simulink model "TIE2019Simulation"  (R2016b)
settings: Solver=FixedStepAuto  StartTime=0.0  StopTime=100  FixedStep=0.01  RelTol=1e-3
InitFcn:
  | Disturbance_rotor_payload_ini;
StopFcn:
  | PlotResults;
values from neighbouring files (symbols this model uses):
  b1 = 220    [Disturbance_rotor_payload_ini.m]
  b2 = 110    [Disturbance_rotor_payload_ini.m]
  c_v = 1    [Disturbance_rotor_payload_ini.m]
  c_x = 1    [Disturbance_rotor_payload_ini.m]
  delta_W = 0*n    [Disturbance_rotor_payload_ini.m]
  g_I = [0 0 9.8]'    [Disturbance_rotor_payload_ini.m]
  invJ_B1 = inv(J)    [Disturbance_rotor_payload_ini.m]
  J = [2 0.3 -0.5;0.3 1 0.2;-0.5 0.2 3]*10^-2    [Disturbance_rotor_payload_ini.m]
  k = 0.6    [Disturbance_rotor_payload_ini.m]
  k_e = 15    [Disturbance_rotor_payload_ini.m]
  K_omega = 1*eye(3)    [Disturbance_rotor_payload_ini.m]
  K_q = 100    [Disturbance_rotor_payload_ini.m]
  K_R = 1*eye(3)    [Disturbance_rotor_payload_ini.m]
  k_v = 15    [Disturbance_rotor_payload_ini.m]
  L = 2    [Disturbance_rotor_payload_ini.m]
  Lambda_initalB01 = angle2quat(initial_Euler(3),initial_Euler(2),initial_Euler(1))    [Disturbance_rotor_payload_ini.m]
  lambda_p = 0.2    [Disturbance_rotor_payload_ini.m]
  lambda_q = 0.3    [Disturbance_rotor_payload_ini.m]
  lambda_theta = 1    [Disturbance_rotor_payload_ini.m]
  lambda_x = 1/20    (= 0.05)    [Disturbance_rotor_payload_ini.m]
  m_p = 2    [Disturbance_rotor_payload_ini.m]
  m_q = 2    [Disturbance_rotor_payload_ini.m]
  mid_point = (mid_point1+mid_point2)/2    [Disturbance_rotor_payload_ini.m]
  n = [n;0]    [Disturbance_rotor_payload_ini.m]
  n_ = n_/norm(n_)    [Disturbance_rotor_payload_ini.m]
  omega_b01 = [0.1 0.3 0]'    [Disturbance_rotor_payload_ini.m]
  sin_W = -5    [Disturbance_rotor_payload_ini.m]
  U_initial = [y_dot_initial;v_q]    [Disturbance_rotor_payload_ini.m]
  W_0 = (m_p+m_q)*v_q + m_p*B0*y_dot_initial    [Disturbance_rotor_payload_ini.m]
  W_p = [-3 3 -0.5]'    [Disturbance_rotor_payload_ini.m]
  W_q = [-5 4 -0.3]'    [Disturbance_rotor_payload_ini.m]
  waypoint_n = [n1 n2 n3 n4 n5]    [Disturbance_rotor_payload_ini.m]
  waypoint_p = [P1 P2 P3 P4 P5]    [Disturbance_rotor_payload_ini.m]
  waypoint_v = [v1 v2 v3 v4 v5]'    [Disturbance_rotor_payload_ini.m]
  X_initial = [0 0 0]'    [Disturbance_rotor_payload_ini.m]
  y_inital = [0.02 -0.02]'    [Disturbance_rotor_payload_ini.m]
libraries: aerolibtransform2 x4, dspmtrx3 x2, aerolibutil x2, dspinverses x2
(part 1 of 2)
settings Model: Creator=arthus  LastModifiedBy=longh

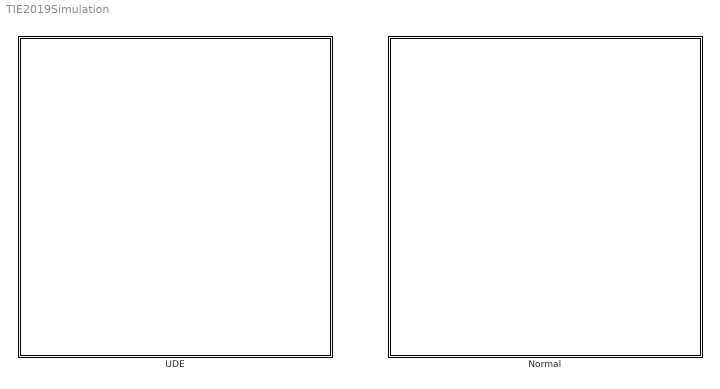
== system TIE2019Simulation ==
  Normal : Subsystem
  UDE : Subsystem
  wires:
  ? -> ?

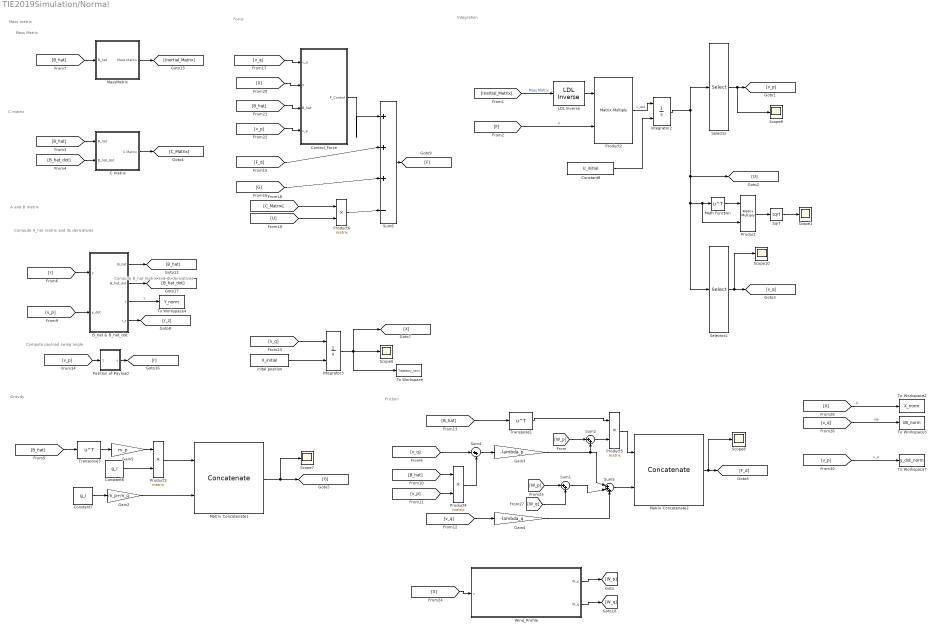
== system TIE2019Simulation/Normal ==
  note: Friction
  note: Gravity
  note: C matrix
  note: Force
  note: A and B matrix
  note: Mass matrix
  note: Mass Matrix
  note: Compute B_hat matrix and its derivatives
  note: Compute A_hat matrix and its derivatives
  note: Integration
  note: Compute payload swing angle
  note: X
  B_hat & B_hat_dot : Subsystem
  C matrix : Subsystem
  Constant6 : Constant  Value=g_I  VectorParams1D=off
  Constant7 : Constant  Value=g_I  VectorParams1D=off
  Constant8 : Constant  Value=U_initial  VectorParams1D=off
  Control_Force : Subsystem
  Gain2 : Gain  Gain=m_p+m_q
  Gain3 : Gain  Gain=-lambda_p
  Gain4 : Gain  Gain=-lambda_q
  Gain5 : Gain  Gain=m_p
  Integrator2 : Integrator  InitialConditionSource=external  InitialCondition=U_initial
  Integrator3 : Integrator  InitialConditionSource=external
  LDL Inverse : dspinverses/LDL Inverse  errmode=Error
  MassMatrix : Subsystem
  Math Function : Math  Operator=transpose  SaturateOnIntegerOverflow=on
  Matrix Concatenate1 : Concatenate  Mode=Multidimensional array
  Matrix Concatenate2 : Concatenate  Mode=Multidimensional array
  Position of Payload : Subsystem
  Product{,3..6} (5 alike) : Product  Multiplication=Matrix(*)
  Product2 : Product  Multiplication=Matrix(*)  RndMeth=Zero
  Scope{1,6..10} (6 alike) : Scope
  Selector : Selector  InputPortWidth=5  IndexOptions=Index vector (dialog)  Indices=[1 2]  OutputSizes=1
  Selector2 : Selector  InputPortWidth=5  IndexOptions=Index vector (dialog)  Indices=[3 4 5]  OutputSizes=1
  Sqrt : Sqrt  SaturateOnIntegerOverflow=on
  Sum1 : Sum  Inputs=|++
  Sum2 : Sum  Inputs=|++
  Sum4 : Sum  Inputs=|++
  Sum5 : Sum  Inputs=|+++
  Sum6 : Sum  Inputs=|+++-
  To Workspace : ToWorkspace  VariableName=Trajectory_norm  SampleTime=-1
  To Workspace2 : ToWorkspace  VariableName=X_norm  SaveFormat=Structure With Time  SampleTime=-1
  To Workspace3 : ToWorkspace  VariableName=VB_norm  SaveFormat=Structure With Time  SampleTime=-1
  To Workspace4 : ToWorkspace  VariableName=Y_norm  SaveFormat=Structure With Time  SampleTime=-1
  To Workspace7 : ToWorkspace  VariableName=y_dot_norm  SaveFormat=Structure With Time  SampleTime=-1
  Transpose1 : Math  Operator=transpose  SaturateOnIntegerOverflow=on
  Transpose3 : Math  Operator=transpose  SaturateOnIntegerOverflow=on
  Wind_Profile : Subsystem
  inital position : Constant  Value=X_initial
  wires:
  MassMatrix/1(Mass Matrix) -> [Inertial_Matrix]
  B_hat & B_hat_dot/2(B_hat_dot) -> [B_hat_dot]
  B_hat & B_hat_dot/1(B_hat) -> [B_hat]
  [r] -> B_hat & B_hat_dot/1(y)
  [v_p] -> B_hat & B_hat_dot/2(y_dot)
  [B_hat] -> MassMatrix/1(B_hat)
  LDL Inverse/1 -> Product2/1
  [Inertial_Matrix] -> LDL Inverse/1  "Mass Matrix"
  [F] -> Product2/2  "F"
  Selector/1 -> Scope9/1, [v_p]
  Product2/1 -> Integrator2/1  "u_dot"
  Integrator2/1 -> Selector/1, [U], Product/2, Math Function/1, Selector2/1
  Selector2/1 -> Scope10/1, [v_q]
  C matrix/1(C Matrix) -> [C_Matrix]
  [B_hat] -> C matrix/1(B_hat)
  [B_hat_dot] -> C matrix/2(B_hat_dot)
  [B_hat] -> Transpose3/1
  Gain5/1 -> Product3/1
  Constant6/1 -> Product3/2
  Transpose3/1 -> Gain5/1
  Product3/1 -> Matrix Concatenate1/1
  Constant7/1 -> Gain2/1
  Gain2/1 -> Matrix Concatenate1/2
  Matrix Concatenate1/1 -> Scope7/1, [G]
  Matrix Concatenate2/1 -> Scope8/1, [F_d]
  Sum5/1 -> Matrix Concatenate2/2
  Sum4/1 -> Gain3/1
  [v_q] -> Sum4/1
  [B_hat] -> Product4/1
  [v_p] -> Product4/2
  Product4/1 -> Sum4/2
  [v_q] -> Gain4/1
  [B_hat] -> Transpose1/1
  Transpose1/1 -> Product5/1
  Product5/1 -> Matrix Concatenate2/1
  Position of Payload/1(y) -> [r]
  [v_p] -> Position of Payload/1(y_dot)
  Sum6/1 -> [F]
  Control_Force/1(F_Control) -> Sum6/1
  [F_d] -> Sum6/2
  [G] -> Sum6/3
  [C_Matrix] -> Product6/1
  [U] -> Product6/2
  Product6/1 -> Sum6/4
  inital position/1 -> Integrator3/2
  [v_q] -> Integrator3/1
  Constant8/1 -> Integrator2/2
  [v_q] -> Control_Force/1(v_q)
  [X] -> Control_Force/2(X)
  B_hat & B_hat_dot/4(r_z) -> [r_z]
  Integrator3/1 -> To Workspace/1, [X], Scope6/1
  Gain4/1 -> Sum5/3
  Sum1/1 -> Sum5/2
  Sum2/1 -> Product5/2
  Gain3/1 -> Sum2/2, Sum5/1
  [B_hat] -> Control_Force/3("B_hat ")
  [v_p] -> Control_Force/4(v_p)
  B_hat & B_hat_dot/3(Y) -> To Workspace4/1  "Y"
  [v_q] -> To Workspace3/1  "VB"
  [X] -> To Workspace2/1
  [v_p] -> To Workspace7/1  "v_p"
  Wind_Profile/1(W_p) -> [W_p]
  [W_p] -> Sum2/1
  [W_q] -> Sum1/2
  [W_p] -> Sum1/1
  Math Function/1 -> Product/1
  Product/1 -> Sqrt/1
  Sqrt/1 -> Scope1/1
  Wind_Profile/2(W_q) -> [W_q]
  [X] -> Wind_Profile/1(x)

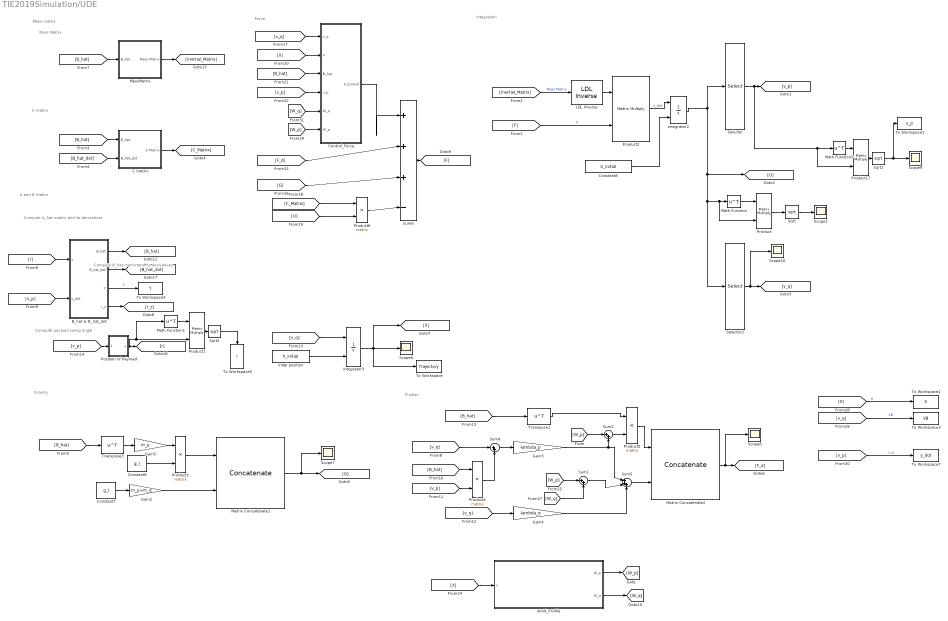
== system TIE2019Simulation/UDE ==
  note: Friction
  note: Gravity
  note: C matrix
  note: Force
  note: A and B matrix
  note: Mass matrix
  note: Mass Matrix
  note: Compute B_hat matrix and its derivatives
  note: Compute A_hat matrix and its derivatives
  note: Integration
  note: Compute payload swing angle
  note: X
  B_hat & B_hat_dot : Subsystem
  C matrix : Subsystem
  Constant6 : Constant  Value=g_I  VectorParams1D=off
  Constant7 : Constant  Value=g_I  VectorParams1D=off
  Constant8 : Constant  Value=U_initial  VectorParams1D=off
  Control_Force : Subsystem
  Gain2 : Gain  Gain=m_p+m_q
  Gain3 : Gain  Gain=-lambda_p
  Gain4 : Gain  Gain=-lambda_q
  Gain5 : Gain  Gain=m_p
  Integrator2 : Integrator  InitialConditionSource=external  InitialCondition=U_initial
  Integrator3 : Integrator  InitialConditionSource=external
  LDL Inverse : dspinverses/LDL Inverse  errmode=Error
  MassMatrix : Subsystem
  Math Function : Math  Operator=transpose  SaturateOnIntegerOverflow=on
  Math Function1 : Math  Operator=transpose  SaturateOnIntegerOverflow=on
  Math Function5 : Math  Operator=transpose  SaturateOnIntegerOverflow=on
  Matrix Concatenate1 : Concatenate  Mode=Multidimensional array
  Matrix Concatenate2 : Concatenate  Mode=Multidimensional array
  Position of Payload : Subsystem
  Product{,1,3..6,17} (7 alike) : Product  Multiplication=Matrix(*)
  Product2 : Product  Multiplication=Matrix(*)  RndMeth=Zero
  Scope{1,6..10} (6 alike) : Scope
  Selector : Selector  InputPortWidth=5  IndexOptions=Index vector (dialog)  Indices=[1 2]  OutputSizes=1
  Selector2 : Selector  InputPortWidth=5  IndexOptions=Index vector (dialog)  Indices=[3 4 5]  OutputSizes=1
  Sqrt : Sqrt  SaturateOnIntegerOverflow=on
  Sqrt1 : Sqrt  SaturateOnIntegerOverflow=on
  Sqrt2 : Sqrt  SaturateOnIntegerOverflow=on
  Sum1 : Sum  Inputs=|++
  Sum2 : Sum  Inputs=|++
  Sum4 : Sum  Inputs=|++
  Sum5 : Sum  Inputs=|+++
  Sum6 : Sum  Inputs=|+++-
  To Workspace : ToWorkspace  VariableName=Trajectory  SampleTime=-1
  To Workspace1 : ToWorkspace  VariableName=v_p  SampleTime=-1
  To Workspace2 : ToWorkspace  VariableName=X  SaveFormat=Structure With Time  SampleTime=-1
  To Workspace3 : ToWorkspace  VariableName=VB  SaveFormat=Structure With Time  SampleTime=-1
  To Workspace4 : ToWorkspace  VariableName=Y  SaveFormat=Structure With Time  SampleTime=-1
  To Workspace5 : ToWorkspace  VariableName=r  SampleTime=-1
  To Workspace7 : ToWorkspace  VariableName=y_dot  SaveFormat=Structure With Time  SampleTime=-1
  Transpose1 : Math  Operator=transpose  SaturateOnIntegerOverflow=on
  Transpose3 : Math  Operator=transpose  SaturateOnIntegerOverflow=on
  Wind_Profile : Subsystem
  inital position : Constant  Value=X_initial
  wires:
  MassMatrix/1(Mass Matrix) -> [Inertial_Matrix]
  B_hat & B_hat_dot/2(B_hat_dot) -> [B_hat_dot]
  B_hat & B_hat_dot/1(B_hat) -> [B_hat]
  [r] -> B_hat & B_hat_dot/1(y)
  [v_p] -> B_hat & B_hat_dot/2(y_dot)
  [B_hat] -> MassMatrix/1(B_hat)
  LDL Inverse/1 -> Product2/1
  [Inertial_Matrix] -> LDL Inverse/1  "Mass Matrix"
  [F] -> Product2/2  "F"
  Product2/1 -> Integrator2/1  "u_dot"
  Integrator2/1 -> Selector/1, [U], Product/2, Math Function/1, Selector2/1
  Selector2/1 -> Scope10/1, [v_q]
  C matrix/1(C Matrix) -> [C_Matrix]
  [B_hat] -> C matrix/1(B_hat)
  [B_hat_dot] -> C matrix/2(B_hat_dot)
  [B_hat] -> Transpose3/1
  Gain5/1 -> Product3/1
  Constant6/1 -> Product3/2
  Transpose3/1 -> Gain5/1
  Product3/1 -> Matrix Concatenate1/1
  Constant7/1 -> Gain2/1
  Gain2/1 -> Matrix Concatenate1/2
  Matrix Concatenate1/1 -> Scope7/1, [G]
  Matrix Concatenate2/1 -> Scope8/1, [F_d]
  Sum5/1 -> Matrix Concatenate2/2
  Sum4/1 -> Gain3/1
  [v_q] -> Sum4/1
  [B_hat] -> Product4/1
  [v_p] -> Product4/2
  Product4/1 -> Sum4/2
  [v_q] -> Gain4/1
  [B_hat] -> Transpose1/1
  Transpose1/1 -> Product5/1
  Product5/1 -> Matrix Concatenate2/1
  Position of Payload/1(y) -> Math Function1/1, Product1/2, [r]
  [v_p] -> Position of Payload/1(y_dot)
  Sum6/1 -> [F]
  Control_Force/1(F_Control) -> Sum6/1
  [F_d] -> Sum6/2
  [G] -> Sum6/3
  [C_Matrix] -> Product6/1
  [U] -> Product6/2
  Product6/1 -> Sum6/4
  inital position/1 -> Integrator3/2
  [v_q] -> Integrator3/1
  Constant8/1 -> Integrator2/2
  [v_q] -> Control_Force/1(v_q)
  [X] -> Control_Force/2(X)
  B_hat & B_hat_dot/4(r_z) -> [r_z]
  Integrator3/1 -> To Workspace/1, [X], Scope6/1
  Gain4/1 -> Sum5/3
  Sum1/1 -> Sum5/2
  Sum2/1 -> Product5/2
  Gain3/1 -> Sum2/2, Sum5/1
  [B_hat] -> Control_Force/3("B_hat ")
  [v_p] -> Control_Force/4(v_p)
  B_hat & B_hat_dot/3(Y) -> To Workspace4/1  "Y"
  [v_q] -> To Workspace3/1  "VB"
  [X] -> To Workspace2/1
  [v_p] -> To Workspace7/1  "v_p"
  Wind_Profile/1(W_p) -> [W_p]
  [W_p] -> Sum2/1
  [W_q] -> Sum1/2
  [W_p] -> Sum1/1
  Math Function/1 -> Product/1
  Product/1 -> Sqrt/1
  Sqrt/1 -> Scope1/1
  Wind_Profile/2(W_q) -> [W_q]
  [X] -> Wind_Profile/1(x)
  Selector/1 -> Math Function5/1, Product17/2, [v_p]
  Math Function5/1 -> Product17/1
  Product17/1 -> Sqrt1/1
  Sqrt1/1 -> To Workspace1/1, Scope9/1
  [W_p] -> Control_Force/6(W_p)
  [W_q] -> Control_Force/5(W_q)
  Math Function1/1 -> Product1/1
  Product1/1 -> Sqrt2/1
  Sqrt2/1 -> To Workspace5/1

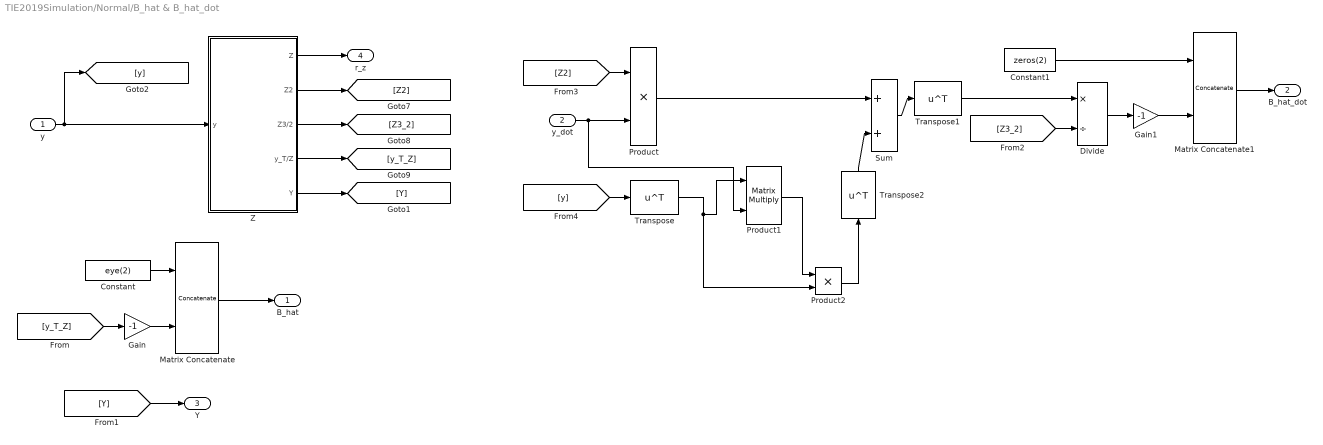
== system TIE2019Simulation/Normal/B_hat & B_hat_dot ==
  y : Inport
  y_dot : Inport  Port=2
  Constant : Constant  Value=eye(2)
  Constant1 : Constant  Value=zeros(2)
  Divide : Product  Inputs=*/
  Gain : Gain  Gain=-1
  Gain1 : Gain  Gain=-1
  Matrix Concatenate : Concatenate  Mode=Multidimensional array
  Matrix Concatenate1 : Concatenate  Mode=Multidimensional array
  Product : Product  RndMeth=Zero
  Product1 : Product  Multiplication=Matrix(*)  RndMeth=Zero
  Product2 : Product  RndMeth=Zero
  Sum : Sum
  Transpose : Math  Operator=transpose  SaturateOnIntegerOverflow=on
  Transpose1 : Math  Operator=transpose  SaturateOnIntegerOverflow=on
  Transpose2 : Math  Operator=transpose  SaturateOnIntegerOverflow=on
  Z : Subsystem
  B_hat : Outport
  B_hat_dot : Outport  Port=2
  Y : Outport  Port=3
  r_z : Outport  Port=4
  wires:
  y_dot/1 -> Product/2, Product1/2
  y/1 -> Z/1(y), [y]
  Matrix Concatenate/1 -> B_hat/1
  Matrix Concatenate1/1 -> B_hat_dot/1
  Z/1(Z) -> r_z/1
  Z/2(Z2) -> [Z2]
  Z/3(Z3/2) -> [Z3_2]
  Z/4(y_T/Z) -> [y_T_Z]
  [y_T_Z] -> Gain/1
  Constant/1 -> Matrix Concatenate/1
  Gain/1 -> Matrix Concatenate/2
  Z/5(Y) -> [Y]
  [Y] -> Y/1
  Constant1/1 -> Matrix Concatenate1/1
  [Z3_2] -> Divide/2
  Sum/1 -> Transpose1/1
  [Z2] -> Product/1
  [y] -> Transpose/1
  Transpose/1 -> Product1/1, Product2/2
  Product1/1 -> Product2/1
  Divide/1 -> Gain1/1
  Gain1/1 -> Matrix Concatenate1/2
  Product2/1 -> Transpose2/1
  Product/1 -> Sum/1
  Transpose1/1 -> Divide/1
  Transpose2/1 -> Sum/2

== system TIE2019Simulation/Normal/C matrix ==
  B_hat : Inport
  B_hat_dot : Inport  Port=2
  Constant : Constant  Value=[zeros(2,3);zeros(3)]  VectorParams1D=off
  Gain4 : Gain  Gain=m_p
  Gain5 : Gain  Gain=m_p
  Matrix Concatenate : Concatenate  Mode=Multidimensional array  ConcatenateDimension=2
  Matrix Concatenate1 : Concatenate  Mode=Multidimensional array
  Product1 : Product  Multiplication=Matrix(*)
  Transpose3 : Math  Operator=transpose  SaturateOnIntegerOverflow=on
  C Matrix : Outport
  wires:
  Matrix Concatenate/1 -> C Matrix/1
  Matrix Concatenate1/1 -> Matrix Concatenate/1
  Constant/1 -> Matrix Concatenate/2
  B_hat/1 -> Transpose3/1
  Transpose3/1 -> [B_hatT]
  Gain5/1 -> Matrix Concatenate1/1
  [B_hatT] -> Product1/1
  B_hat_dot/1 -> Gain4/1, Product1/2
  Product1/1 -> Gain5/1
  Gain4/1 -> Matrix Concatenate1/2

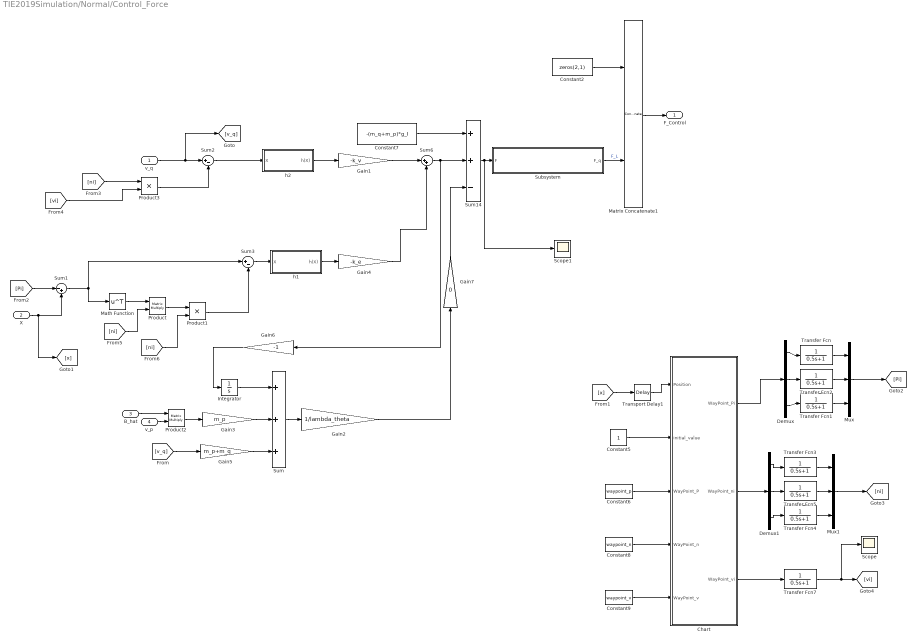
== system TIE2019Simulation/Normal/Control_Force ==
  v_q : Inport
  X : Inport  Port=2
  "B_hat " : Inport  Port=3
  v_p : Inport  Port=4
  Chart : Stateflow chart  TreatAsAtomicUnit=on
  Constant2 : Constant  Value=zeros(2,1)
  Constant5 : Constant
  Constant6 : Constant  Value=waypoint_p
  Constant7 : Constant  Value=-(m_q+m_p)*g_I  VectorParams1D=off
  Constant8 : Constant  Value=waypoint_n
  Constant9 : Constant  Value=waypoint_v
  Demux : Demux  Outputs=3
  Demux1 : Demux  Outputs=3
  Gain1 : Gain  Gain=-k_v
  Gain2 : Gain  Gain=1/lambda_theta
  Gain3 : Gain  Gain=m_p
  Gain4 : Gain  Gain=-k_e
  Gain5 : Gain  Gain=m_p+m_q
  Gain6 : Gain  Gain=-1
  Gain7 : Gain  Gain=0
  Integrator : Integrator
  Math Function : Math  Operator=transpose  SaturateOnIntegerOverflow=on
  Matrix Concatenate1 : Concatenate  Mode=Multidimensional array
  Mux : Mux  Inputs=3
  Mux1 : Mux  Inputs=3
  Product : Product  Multiplication=Matrix(*)
  Product1 : Product
  Product2 : Product  Multiplication=Matrix(*)
  Product3 : Product
  Scope : Scope
  Scope1 : Scope
  Subsystem : Subsystem
  Sum : Sum  Inputs=+++
  Sum1 : Sum  Inputs=|-+
  Sum14 : Sum  Inputs=++-
  Sum2 : Sum  Inputs=|+-
  Sum3 : Sum  Inputs=|+-
  Sum6 : Sum  Inputs=|++
  Transfer Fcn{,1..5,7} (7 alike) : TransferFcn  Denominator=[0.5 1]
  Transport Delay1 : TransportDelay  DelayTime=0.3
  h1 : Subsystem
  h2 : Subsystem
  F_Control : Outport
  wires:
  Constant2/1 -> Matrix Concatenate1/1
  X/1 -> [x], Sum1/2
  v_q/1 -> [v_q], Sum2/1
  Sum14/1 -> Scope1/1, Subsystem/1(F)
  [ni] -> Product3/1
  [Pi] -> Sum1/1
  Product3/1 -> Sum2/2
  h1/1(h(X)) -> Gain4/1
  Gain4/1 -> Sum6/2
  Sum1/1 -> Sum3/1, Math Function/1
  Math Function/1 -> Product/1
  [ni] -> Product/2
  Product/1 -> Product1/1
  [ni] -> Product1/2
  Product1/1 -> Sum3/2
  Gain1/1 -> Sum6/1
  h2/1(h(X)) -> Gain1/1
  Sum6/1 -> Gain6/1, Sum14/2
  Constant7/1 -> Sum14/1
  Gain2/1 -> Gain7/1
  Sum/1 -> Gain2/1
  "B_hat "/1 -> Product2/1
  v_p/1 -> Product2/2
  Product2/1 -> Gain3/1
  [v_q] -> Gain5/1
  Gain3/1 -> Sum/2
  Gain5/1 -> Sum/3
  Integrator/1 -> Sum/1
  Gain6/1 -> Integrator/1
  Matrix Concatenate1/1 -> F_Control/1
  Gain7/1 -> Sum14/3
  Subsystem/1(F_q) -> Matrix Concatenate1/2  "F_L"
  Constant5/1 -> Chart/2(initial_value)
  [x] -> Transport Delay1/1
  Constant6/1 -> Chart/3(WayPoint_P)
  Constant8/1 -> Chart/4(WayPoint_n)
  Constant9/1 -> Chart/5(WayPoint_v)
  [vi] -> Product3/2
  Transport Delay1/1 -> Chart/1(Position)
  Demux/3 -> Transfer Fcn1/1
  Transfer Fcn1/1 -> Mux/3
  Demux/2 -> Transfer Fcn2/1
  Transfer Fcn2/1 -> Mux/2
  Demux/1 -> Transfer Fcn/1
  Transfer Fcn/1 -> Mux/1
  Mux/1 -> [Pi]
  Chart/1(WayPoint_Pi) -> Demux/1
  Demux1/3 -> Transfer Fcn4/1
  Transfer Fcn4/1 -> Mux1/3
  Demux1/2 -> Transfer Fcn5/1
  Transfer Fcn5/1 -> Mux1/2
  Demux1/1 -> Transfer Fcn3/1
  Transfer Fcn3/1 -> Mux1/1
  Mux1/1 -> [ni]
  Chart/2(WayPoint_ni) -> Demux1/1
  Chart/3(WayPoint_vi) -> Transfer Fcn7/1
  Transfer Fcn7/1 -> Scope/1, [vi]
  Sum2/1 -> h2/1(X)
  Sum3/1 -> h1/1(X)

== system TIE2019Simulation/Normal/MassMatrix ==
  B_hat : Inport
  Constant : Constant  Value=(m_q+m_p)*eye(3)
  Gain1 : Gain  Gain=m_p
  Gain2 : Gain  Gain=m_p
  Gain3 : Gain  Gain=m_p
  Matrix Concatenate : Concatenate  Mode=Multidimensional array  ConcatenateDimension=2
  Matrix Concatenate1 : Concatenate  Mode=Multidimensional array
  Matrix Concatenate2 : Concatenate  Mode=Multidimensional array
  Product : Product  Multiplication=Matrix(*)
  Transpose3 : Math  Operator=transpose  SaturateOnIntegerOverflow=on
  Mass Matrix : Outport
  wires:
  Matrix Concatenate/1 -> Mass Matrix/1
  Matrix Concatenate1/1 -> Matrix Concatenate/1
  Matrix Concatenate2/1 -> Matrix Concatenate/2
  B_hat/1 -> [B_hat], Transpose3/1
  Transpose3/1 -> [B_hatT]
  [B_hatT] -> Product/1
  [B_hat] -> Product/2
  Product/1 -> Gain1/1
  Gain1/1 -> Matrix Concatenate1/1
  Gain2/1 -> Matrix Concatenate1/2
  [B_hat] -> Gain2/1
  Constant/1 -> Matrix Concatenate2/2
  [B_hatT] -> Gain3/1
  Gain3/1 -> Matrix Concatenate2/1

== system TIE2019Simulation/Normal/Position of Payload ==
  y_dot : Inport
  Integrator : Integrator  InitialConditionSource=external
  inital position : Constant  Value=y_inital  VectorParams1D=off
  y : Outport
  wires:
  Integrator/1 -> y/1
  y_dot/1 -> Integrator/1
  inital position/1 -> Integrator/2

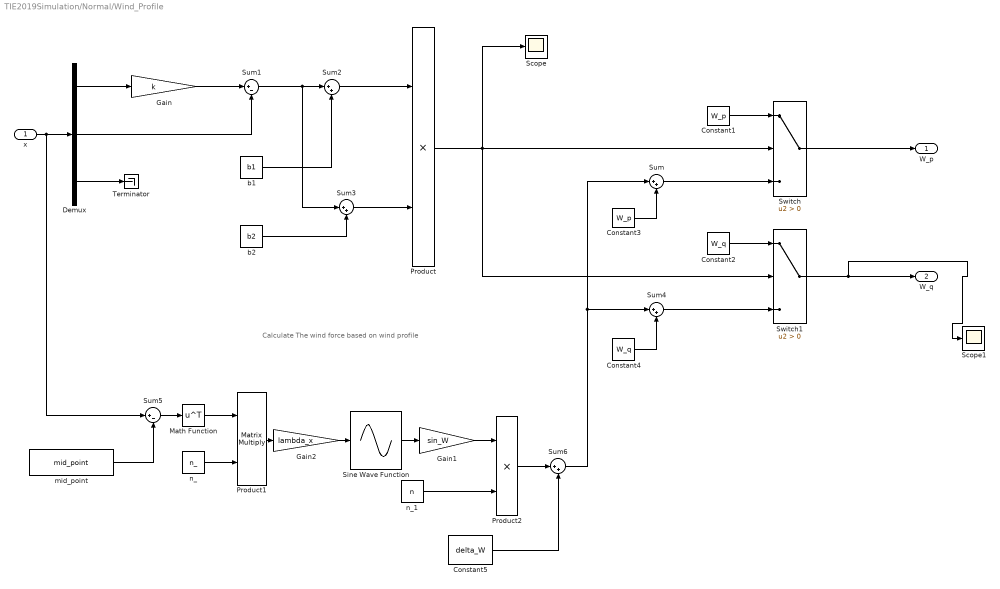
== system TIE2019Simulation/Normal/Wind_Profile ==
  note: Calculate The wind force based on wind profile
  x : Inport
  Constant1 : Constant  Value=W_p
  Constant2 : Constant  Value=W_q
  Constant3 : Constant  Value=W_p
  Constant4 : Constant  Value=W_q
  Constant5 : Constant  Value=delta_W
  Demux : Demux  Outputs=3
  Gain : Gain  Gain=k
  Gain1 : Gain  Gain=sin_W
  Gain2 : Gain  Gain=lambda_x
  Math Function : Math  Operator=transpose  SaturateOnIntegerOverflow=on
  Product : Product
  Product1 : Product  Multiplication=Matrix(*)
  Product2 : Product
  Scope : Scope
  Scope1 : Scope
  Sine Wave Function : Sin  TimeSource=Use external signal  SampleTime=0
  Sum{,2..4,6} (5 alike) : Sum  Inputs=|++
  Sum1 : Sum  Inputs=|+-
  Sum5 : Sum  Inputs=|+-
  Switch : Switch  Criteria=u2 > Threshold
  Switch1 : Switch  Criteria=u2 > Threshold
  Terminator : Terminator
  b1 : Constant  Value=b1
  b2 : Constant  Value=b2
  "mid_point " : Constant  Value=mid_point  VectorParams1D=off
  n_ : Constant  Value=n_
  n_1 : Constant  Value=n
  W_p : Outport
  W_q : Outport  Port=2
  wires:
  Demux/3 -> Terminator/1
  Demux/1 -> Gain/1
  Demux/2 -> Sum1/2
  Gain/1 -> Sum1/1
  Sum1/1 -> Sum3/1, Sum2/1
  b1/1 -> Sum2/2
  b2/1 -> Sum3/2
  Sum2/1 -> Product/1
  Sum3/1 -> Product/2
  Product/1 -> Scope/1, Switch1/2, Switch/2
  Constant2/1 -> Switch1/1
  Constant1/1 -> Switch/1
  Switch/1 -> W_p/1
  Switch1/1 -> Scope1/1, W_q/1
  Sine Wave Function/1 -> Gain1/1
  Sum/1 -> Switch/3
  Sum4/1 -> Switch1/3
  Constant3/1 -> Sum/2
  Constant4/1 -> Sum4/2
  x/1 -> Sum5/1, Demux/1
  "mid_point "/1 -> Sum5/2
  Sum5/1 -> Math Function/1
  Math Function/1 -> Product1/1
  n_/1 -> Product1/2
  Product1/1 -> Gain2/1
  Gain1/1 -> Product2/1
  n_1/1 -> Product2/2
  Gain2/1 -> Sine Wave Function/1
  Product2/1 -> Sum6/1
  Sum6/1 -> Sum4/1, Sum/1
  Constant5/1 -> Sum6/2

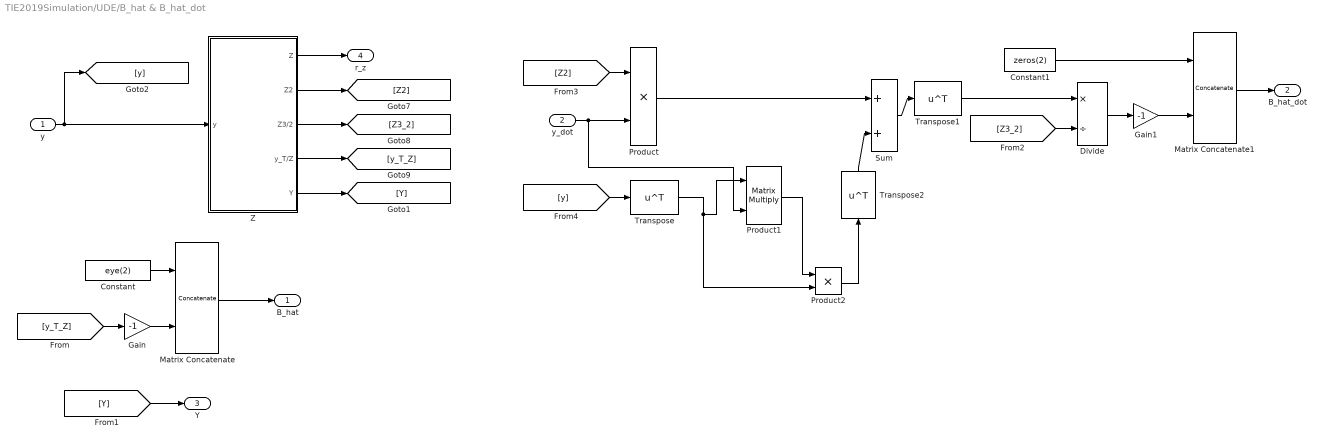
== system TIE2019Simulation/UDE/B_hat & B_hat_dot ==
  y : Inport
  y_dot : Inport  Port=2
  Constant : Constant  Value=eye(2)
  Constant1 : Constant  Value=zeros(2)
  Divide : Product  Inputs=*/
  Gain : Gain  Gain=-1
  Gain1 : Gain  Gain=-1
  Matrix Concatenate : Concatenate  Mode=Multidimensional array
  Matrix Concatenate1 : Concatenate  Mode=Multidimensional array
  Product : Product  RndMeth=Zero
  Product1 : Product  Multiplication=Matrix(*)  RndMeth=Zero
  Product2 : Product  RndMeth=Zero
  Sum : Sum
  Transpose : Math  Operator=transpose  SaturateOnIntegerOverflow=on
  Transpose1 : Math  Operator=transpose  SaturateOnIntegerOverflow=on
  Transpose2 : Math  Operator=transpose  SaturateOnIntegerOverflow=on
  Z : Subsystem
  B_hat : Outport
  B_hat_dot : Outport  Port=2
  Y : Outport  Port=3
  r_z : Outport  Port=4
  wires:
  y_dot/1 -> Product/2, Product1/2
  y/1 -> Z/1(y), [y]
  Matrix Concatenate/1 -> B_hat/1
  Matrix Concatenate1/1 -> B_hat_dot/1
  Z/1(Z) -> r_z/1
  Z/2(Z2) -> [Z2]
  Z/3(Z3/2) -> [Z3_2]
  Z/4(y_T/Z) -> [y_T_Z]
  [y_T_Z] -> Gain/1
  Constant/1 -> Matrix Concatenate/1
  Gain/1 -> Matrix Concatenate/2
  Z/5(Y) -> [Y]
  [Y] -> Y/1
  Constant1/1 -> Matrix Concatenate1/1
  [Z3_2] -> Divide/2
  Sum/1 -> Transpose1/1
  [Z2] -> Product/1
  [y] -> Transpose/1
  Transpose/1 -> Product1/1, Product2/2
  Product1/1 -> Product2/1
  Divide/1 -> Gain1/1
  Gain1/1 -> Matrix Concatenate1/2
  Product2/1 -> Transpose2/1
  Product/1 -> Sum/1
  Transpose1/1 -> Divide/1
  Transpose2/1 -> Sum/2

== system TIE2019Simulation/UDE/C matrix ==
  B_hat : Inport
  B_hat_dot : Inport  Port=2
  Constant : Constant  Value=[zeros(2,3);zeros(3)]  VectorParams1D=off
  Gain4 : Gain  Gain=m_p
  Gain5 : Gain  Gain=m_p
  Matrix Concatenate : Concatenate  Mode=Multidimensional array  ConcatenateDimension=2
  Matrix Concatenate1 : Concatenate  Mode=Multidimensional array
  Product1 : Product  Multiplication=Matrix(*)
  Transpose3 : Math  Operator=transpose  SaturateOnIntegerOverflow=on
  C Matrix : Outport
  wires:
  Matrix Concatenate/1 -> C Matrix/1
  Matrix Concatenate1/1 -> Matrix Concatenate/1
  Constant/1 -> Matrix Concatenate/2
  B_hat/1 -> Transpose3/1
  Transpose3/1 -> [B_hatT]
  Gain5/1 -> Matrix Concatenate1/1
  [B_hatT] -> Product1/1
  B_hat_dot/1 -> Gain4/1, Product1/2
  Product1/1 -> Gain5/1
  Gain4/1 -> Matrix Concatenate1/2

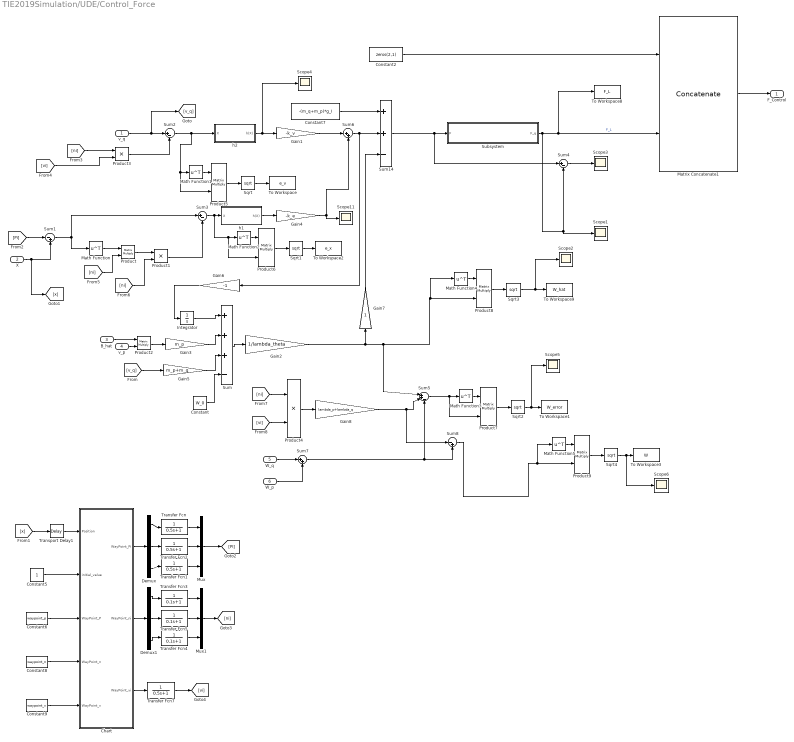
== system TIE2019Simulation/UDE/Control_Force ==
  v_q : Inport
  X : Inport  Port=2
  "B_hat " : Inport  Port=3
  v_p : Inport  Port=4
  W_q : Inport  Port=5
  W_p : Inport  Port=6
  Chart : Stateflow chart  TreatAsAtomicUnit=on
  Constant : Constant  Value=W_0  VectorParams1D=off
  Constant2 : Constant  Value=zeros(2,1)
  Constant5 : Constant
  Constant6 : Constant  Value=waypoint_p
  Constant7 : Constant  Value=-(m_q+m_p)*g_I  VectorParams1D=off
  Constant8 : Constant  Value=waypoint_n
  Constant9 : Constant  Value=waypoint_v
  Demux : Demux  Outputs=3
  Demux1 : Demux  Outputs=3
  Gain1 : Gain  Gain=-k_v
  Gain2 : Gain  Gain=1/lambda_theta
  Gain3 : Gain  Gain=m_p
  Gain4 : Gain  Gain=-k_e
  Gain5 : Gain  Gain=m_p+m_q
  Gain6 : Gain  Gain=-1
  Gain7 : Gain
  Gain8 : Gain  Gain=lambda_p+lambda_q
  Integrator : Integrator
  Math Function{,1..5} (6 alike) : Math  Operator=transpose  SaturateOnIntegerOverflow=on
  Matrix Concatenate1 : Concatenate  Mode=Multidimensional array
  Mux : Mux  Inputs=3
  Mux1 : Mux  Inputs=3
  Product{,2,5..9} (7 alike) : Product  Multiplication=Matrix(*)
  Product1 : Product
  Product3 : Product
  Product4 : Product
  Scope{1..6,11} (7 alike) : Scope
  Sqrt{,1..4} (5 alike) : Sqrt  SaturateOnIntegerOverflow=on
  Subsystem : Subsystem
  Sum : Sum  Inputs=+++-
  Sum1 : Sum  Inputs=|-+
  Sum14 : Sum  Inputs=++-
  Sum2 : Sum  Inputs=|+-
  Sum3 : Sum  Inputs=|+-
  Sum4 : Sum  Inputs=|+-
  Sum5 : Sum  Inputs=|++-
  Sum6 : Sum  Inputs=|++
  Sum7 : Sum  Inputs=|++
  Sum8 : Sum  Inputs=|-+
  To Workspace : ToWorkspace  VariableName=e_v  SampleTime=-1
  To Workspace1 : ToWorkspace  VariableName=W_error  SaveFormat=Structure With Time  SampleTime=-1
  To Workspace2 : ToWorkspace  VariableName=e_x  SampleTime=-1
  To Workspace3 : ToWorkspace  VariableName=W  SaveFormat=Structure With Time  SampleTime=-1
  To Workspace8 : ToWorkspace  VariableName=F_L  SaveFormat=Structure With Time  SampleTime=-1
  To Workspace9 : ToWorkspace  VariableName=W_hat  SaveFormat=Structure With Time  SampleTime=-1
  Transfer Fcn{,1..2,7} (4 alike) : TransferFcn  Denominator=[0.5 1]
  Transfer Fcn3 : TransferFcn  Denominator=[0.1 1]
  Transfer Fcn4 : TransferFcn  Denominator=[0.1 1]
  Transfer Fcn5 : TransferFcn  Denominator=[0.1 1]
  Transport Delay1 : TransportDelay  DelayTime=0.3
  h1 : Subsystem
  h2 : Subsystem
  F_Control : Outport
  wires:
  Constant2/1 -> Matrix Concatenate1/1
  X/1 -> [x], Sum1/2
  v_q/1 -> [v_q], Sum2/1
  Sum14/1 -> Subsystem/1(F), Sum4/1
  [ni] -> Product3/1
  [Pi] -> Sum1/1
  Product3/1 -> Sum2/2
  h1/1(h(X)) -> Gain4/1
  Gain4/1 -> Sum6/2, Scope11/1
  Sum1/1 -> Sum3/1, Math Function/1
  Math Function/1 -> Product/1
  [ni] -> Product/2
  Product/1 -> Product1/1
  [ni] -> Product1/2
  Product1/1 -> Sum3/2
  Gain1/1 -> Sum6/1
  h2/1(h(X)) -> Scope4/1, Gain1/1
  Sum6/1 -> Gain6/1, Sum14/2
  Constant7/1 -> Sum14/1
  Sum/1 -> Gain2/1
  "B_hat "/1 -> Product2/1
  v_p/1 -> Product2/2
  Product2/1 -> Gain3/1
  [v_q] -> Gain5/1
  Gain3/1 -> Sum/2
  Gain5/1 -> Sum/3
  Integrator/1 -> Sum/1
  Gain6/1 -> Integrator/1
  Matrix Concatenate1/1 -> F_Control/1
  Gain7/1 -> Sum14/3
  Subsystem/1(F_q) -> Scope1/1, Sum4/2, To Workspace8/1, Matrix Concatenate1/2  "F_L"
  Sum4/1 -> Scope3/1
  Constant5/1 -> Chart/2(initial_value)
  [x] -> Transport Delay1/1
  Constant6/1 -> Chart/3(WayPoint_P)
  Constant8/1 -> Chart/4(WayPoint_n)
  Constant9/1 -> Chart/5(WayPoint_v)
  [vi] -> Product3/2
  Transport Delay1/1 -> Chart/1(Position)
  Demux/3 -> Transfer Fcn1/1
  Transfer Fcn1/1 -> Mux/3
  Demux/2 -> Transfer Fcn2/1
  Transfer Fcn2/1 -> Mux/2
  Demux/1 -> Transfer Fcn/1
  Transfer Fcn/1 -> Mux/1
  Mux/1 -> [Pi]
  Chart/1(WayPoint_Pi) -> Demux/1
  Demux1/3 -> Transfer Fcn4/1
  Transfer Fcn4/1 -> Mux1/3
  Demux1/2 -> Transfer Fcn5/1
  Transfer Fcn5/1 -> Mux1/2
  Demux1/1 -> Transfer Fcn3/1
  Transfer Fcn3/1 -> Mux1/1
  Mux1/1 -> [ni]
  Chart/2(WayPoint_ni) -> Demux1/1
  Chart/3(WayPoint_vi) -> Transfer Fcn7/1
  Transfer Fcn7/1 -> [vi]
  [ni] -> Product4/1
  Product4/1 -> Gain8/1
  [vi] -> Product4/2
  Gain8/1 -> Sum8/1, Sum5/2
  Sum7/1 -> Sum8/2, Sum5/3
  Sum2/1 -> Product5/2, Math Function1/1, h2/1(X)
  Math Function1/1 -> Product5/1
  Product5/1 -> Sqrt/1
  Sqrt/1 -> To Workspace/1
  Sum3/1 -> Product6/2, Math Function2/1, h1/1(X)
  Math Function2/1 -> Product6/1
  Product6/1 -> Sqrt1/1
  Sum5/1 -> Product7/2, Math Function3/1
  Math Function3/1 -> Product7/1
  Product7/1 -> Sqrt2/1
  Sqrt2/1 -> Scope5/1, To Workspace1/1
  Sqrt1/1 -> To Workspace2/1
  W_q/1 -> Sum7/1
  W_p/1 -> Sum7/2
  Gain2/1 -> Math Function4/1, Product8/2, Sum5/1, Gain7/1
  Math Function4/1 -> Product8/1
  Product8/1 -> Sqrt3/1
  Sqrt3/1 -> Scope2/1, To Workspace9/1
  Sum8/1 -> Math Function5/1, Product9/2
  Math Function5/1 -> Product9/1
  Product9/1 -> Sqrt4/1
  Sqrt4/1 -> Scope6/1, To Workspace3/1
  Constant/1 -> Sum/4

== system TIE2019Simulation/UDE/MassMatrix ==
  B_hat : Inport
  Constant : Constant  Value=(m_q+m_p)*eye(3)
  Gain1 : Gain  Gain=m_p
  Gain2 : Gain  Gain=m_p
  Gain3 : Gain  Gain=m_p
  Matrix Concatenate : Concatenate  Mode=Multidimensional array  ConcatenateDimension=2
  Matrix Concatenate1 : Concatenate  Mode=Multidimensional array
  Matrix Concatenate2 : Concatenate  Mode=Multidimensional array
  Product : Product  Multiplication=Matrix(*)
  Transpose3 : Math  Operator=transpose  SaturateOnIntegerOverflow=on
  Mass Matrix : Outport
  wires:
  Matrix Concatenate/1 -> Mass Matrix/1
  Matrix Concatenate1/1 -> Matrix Concatenate/1
  Matrix Concatenate2/1 -> Matrix Concatenate/2
  B_hat/1 -> [B_hat], Transpose3/1
  Transpose3/1 -> [B_hatT]
  [B_hatT] -> Product/1
  [B_hat] -> Product/2
  Product/1 -> Gain1/1
  Gain1/1 -> Matrix Concatenate1/1
  Gain2/1 -> Matrix Concatenate1/2
  [B_hat] -> Gain2/1
  Constant/1 -> Matrix Concatenate2/2
  [B_hatT] -> Gain3/1
  Gain3/1 -> Matrix Concatenate2/1

== system TIE2019Simulation/UDE/Position of Payload ==
  y_dot : Inport
  Integrator : Integrator  InitialConditionSource=external
  inital position : Constant  Value=y_inital  VectorParams1D=off
  y : Outport
  wires:
  Integrator/1 -> y/1
  y_dot/1 -> Integrator/1
  inital position/1 -> Integrator/2

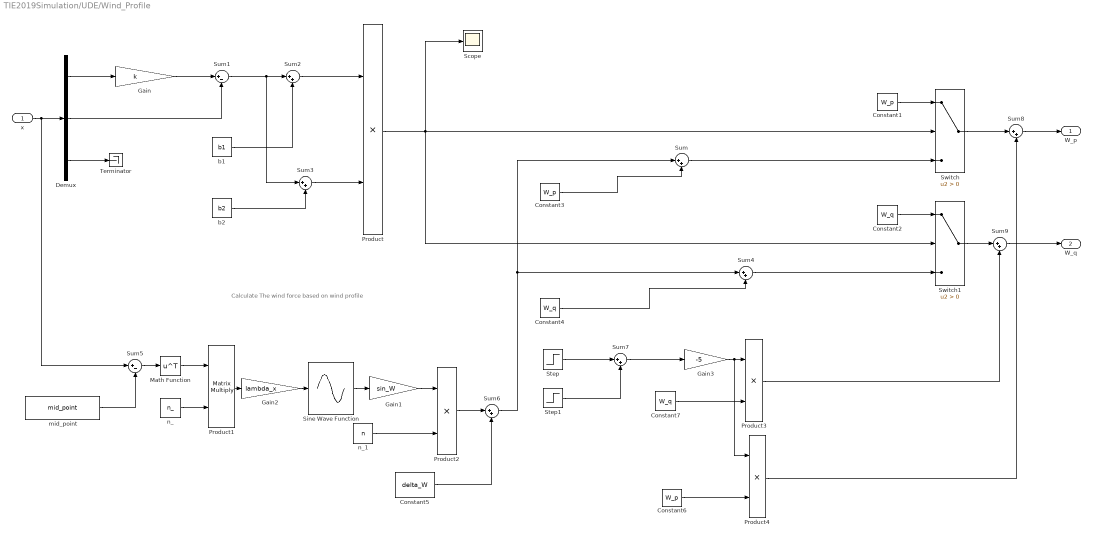
== system TIE2019Simulation/UDE/Wind_Profile ==
  note: Calculate The wind force based on wind profile
  x : Inport
  Constant1 : Constant  Value=W_p
  Constant2 : Constant  Value=W_q
  Constant3 : Constant  Value=W_p
  Constant4 : Constant  Value=W_q
  Constant5 : Constant  Value=delta_W
  Constant6 : Constant  Value=W_p
  Constant7 : Constant  Value=W_q
  Demux : Demux  Outputs=3
  Gain : Gain  Gain=k
  Gain1 : Gain  Gain=sin_W
  Gain2 : Gain  Gain=lambda_x
  Gain3 : Gain  Gain=-5
  Math Function : Math  Operator=transpose  SaturateOnIntegerOverflow=on
  Product{,2..4} (4 alike) : Product
  Product1 : Product  Multiplication=Matrix(*)
  Scope : Scope
  Sine Wave Function : Sin  TimeSource=Use external signal  SampleTime=0
  Step : Step  Time=65  SampleTime=0
  Step1 : Step  Time=67  After=-1  SampleTime=0
  Sum{,2..4,6..9} (8 alike) : Sum  Inputs=|++
  Sum1 : Sum  Inputs=|+-
  Sum5 : Sum  Inputs=|+-
  Switch : Switch  Criteria=u2 > Threshold
  Switch1 : Switch  Criteria=u2 > Threshold
  Terminator : Terminator
  b1 : Constant  Value=b1
  b2 : Constant  Value=b2
  "mid_point " : Constant  Value=mid_point  VectorParams1D=off
  n_ : Constant  Value=n_
  n_1 : Constant  Value=n
  W_p : Outport
  W_q : Outport  Port=2
  wires:
  Demux/3 -> Terminator/1
  Demux/1 -> Gain/1
  Demux/2 -> Sum1/2
  Gain/1 -> Sum1/1
  Sum1/1 -> Sum3/1, Sum2/1
  b1/1 -> Sum2/2
  b2/1 -> Sum3/2
  Sum2/1 -> Product/1
  Sum3/1 -> Product/2
  Product/1 -> Scope/1, Switch1/2, Switch/2
  Constant2/1 -> Switch1/1
  Constant1/1 -> Switch/1
  Sine Wave Function/1 -> Gain1/1
  Sum/1 -> Switch/3
  Sum4/1 -> Switch1/3
  Constant3/1 -> Sum/2
  Constant4/1 -> Sum4/2
  x/1 -> Sum5/1, Demux/1
  "mid_point "/1 -> Sum5/2
  Sum5/1 -> Math Function/1
  Math Function/1 -> Product1/1
  n_/1 -> Product1/2
  Product1/1 -> Gain2/1
  Gain1/1 -> Product2/1
  n_1/1 -> Product2/2
  Gain2/1 -> Sine Wave Function/1
  Product2/1 -> Sum6/1
  Sum6/1 -> Sum4/1, Sum/1
  Constant5/1 -> Sum6/2
  Step/1 -> Sum7/1
  Step1/1 -> Sum7/2
  Gain3/1 -> Product4/1, Product3/1
  Sum7/1 -> Gain3/1
  Constant7/1 -> Product3/2
  Constant6/1 -> Product4/2
  Switch/1 -> Sum8/1
  Sum8/1 -> W_p/1
  Sum9/1 -> W_q/1
  Switch1/1 -> Sum9/1
  Product3/1 -> Sum9/2
  Product4/1 -> Sum8/2

== system TIE2019Simulation/Normal/B_hat & B_hat_dot/Z ==
  y : Inport
  Constant : Constant  Value=L^2  VectorParams1D=off
  Divide : Product  Inputs=*/
  Dot Product : DotProduct  InputSameDT=on  OutDataTypeStr=Inherit: Inherit via internal rule
  Dot Product1 : DotProduct  InputSameDT=on  OutDataTypeStr=Inherit: Inherit via internal rule
  Matrix Concatenate : Concatenate  ConcatenateDimension=2
  Sqrt : Sqrt  SaturateOnIntegerOverflow=on
  Sum : Sum  Inputs=|-+
  Transpose2 : Math  Operator=transpose  SaturateOnIntegerOverflow=on
  Z : Outport
  Z2 : Outport  Port=2
  Z3/2 : Outport  Port=3
  y_T/Z : Outport  Port=4
  Y : Outport  Port=5
  wires:
  y/1 -> Divide/1, Matrix Concatenate/1, Dot Product/2, Dot Product/1
  Constant/1 -> Sum/2
  Dot Product/1 -> Sum/1
  Sum/1 -> Sqrt/1, Z2/1, Dot Product1/2
  Sqrt/1 -> Dot Product1/1, Divide/2, Z/1, Matrix Concatenate/2
  Dot Product1/1 -> Z3/2/1
  Divide/1 -> Transpose2/1
  Transpose2/1 -> y_T/Z/1
  Matrix Concatenate/1 -> Y/1

== system TIE2019Simulation/Normal/Control_Force/Subsystem ==
  F : Inport
  Attitude Dynamics : Subsystem
  Attitude Tracker : Subsystem
  Atttitude Extraction : Subsystem
  Constant : Constant  Value=[0 0 1]'  VectorParams1D=off
  Divide : Product  Inputs=*/
  Dot Product : DotProduct  InputSameDT=on  OutDataTypeStr=Inherit: Inherit via internal rule
  Product : Product  Multiplication=Matrix(*)
  Product1 : Product
  Sqrt : Sqrt  SaturateOnIntegerOverflow=on
  Terminator : Terminator
  Terminator1 : Terminator
  F_q : Outport
  wires:
  F/1 -> Dot Product/2, Dot Product/1, Divide/1
  Constant/1 -> Product/2
  Product/1 -> Product1/2  "n_z"
  Product1/1 -> F_q/1
  Sqrt/1 -> Product1/1, Divide/2
  Dot Product/1 -> Sqrt/1
  Atttitude Extraction/1(R_d) -> Attitude Tracker/1(R_d)
  Atttitude Extraction/2(omega_d) -> Attitude Tracker/2(omega_d)
  Atttitude Extraction/3(omega_d_dot) -> Attitude Tracker/3(omega_d_dot)
  Divide/1 -> Atttitude Extraction/1(n_d)  "n1"
  Attitude Dynamics/4(omega_b) -> Attitude Tracker/5(omega)
  Attitude Dynamics/3(Euler) -> Terminator1/1  "Euler"
  Attitude Dynamics/2(RBI) -> Terminator/1
  Attitude Tracker/1(Torque_in_body_frame) -> Attitude Dynamics/1(MB)  "Mq_b"
  Attitude Dynamics/1(RIB) -> Attitude Tracker/4(R), Product/1  "IRB"

== system TIE2019Simulation/Normal/Control_Force/h1 ==
  X : Inport
  Constant : Constant  Value=c_x
  Divide : Product  Inputs=*/
  Math Function : Math  Operator=transpose  SaturateOnIntegerOverflow=on
  Product : Product  Multiplication=Matrix(*)
  Sum : Sum  Inputs=|++
  h(X) : Outport
  wires:
  X/1 -> Divide/1, Product/2, Math Function/1
  Math Function/1 -> Product/1
  Product/1 -> Sum/1
  Constant/1 -> Sum/2
  Sum/1 -> Divide/2
  Divide/1 -> h(X)/1

== system TIE2019Simulation/Normal/Control_Force/h2 ==
  X : Inport
  Constant : Constant  Value=c_v
  Divide : Product  Inputs=*/
  Math Function : Math  Operator=transpose  SaturateOnIntegerOverflow=on
  Product : Product  Multiplication=Matrix(*)
  Sum : Sum  Inputs=|++
  h(X) : Outport
  wires:
  X/1 -> Divide/1, Product/2, Math Function/1
  Math Function/1 -> Product/1
  Product/1 -> Sum/1
  Constant/1 -> Sum/2
  Sum/1 -> Divide/2
  Divide/1 -> h(X)/1

== system TIE2019Simulation/UDE/B_hat & B_hat_dot/Z ==
  y : Inport
  Constant : Constant  Value=L^2  VectorParams1D=off
  Divide : Product  Inputs=*/
  Dot Product : DotProduct  InputSameDT=on  OutDataTypeStr=Inherit: Inherit via internal rule
  Dot Product1 : DotProduct  InputSameDT=on  OutDataTypeStr=Inherit: Inherit via internal rule
  Matrix Concatenate : Concatenate  ConcatenateDimension=2
  Sqrt : Sqrt  SaturateOnIntegerOverflow=on
  Sum : Sum  Inputs=|-+
  Transpose2 : Math  Operator=transpose  SaturateOnIntegerOverflow=on
  Z : Outport
  Z2 : Outport  Port=2
  Z3/2 : Outport  Port=3
  y_T/Z : Outport  Port=4
  Y : Outport  Port=5
  wires:
  y/1 -> Divide/1, Matrix Concatenate/1, Dot Product/2, Dot Product/1
  Constant/1 -> Sum/2
  Dot Product/1 -> Sum/1
  Sum/1 -> Sqrt/1, Z2/1, Dot Product1/2
  Sqrt/1 -> Dot Product1/1, Divide/2, Z/1, Matrix Concatenate/2
  Dot Product1/1 -> Z3/2/1
  Divide/1 -> Transpose2/1
  Transpose2/1 -> y_T/Z/1
  Matrix Concatenate/1 -> Y/1

== system TIE2019Simulation/UDE/Control_Force/Subsystem ==
  F : Inport
  Attitude Dynamics : Subsystem
  Attitude Tracker : Subsystem
  Atttitude Extraction : Subsystem
  Constant : Constant  Value=[0 0 1]'  VectorParams1D=off
  Divide : Product  Inputs=*/
  Dot Product : DotProduct  InputSameDT=on  OutDataTypeStr=Inherit: Inherit via internal rule
  Product : Product  Multiplication=Matrix(*)
  Product1 : Product
  Sqrt : Sqrt  SaturateOnIntegerOverflow=on
  Terminator : Terminator
  To Workspace1 : ToWorkspace  VariableName=Euler  SaveFormat=Structure With Time  SampleTime=-1
  To Workspace2 : ToWorkspace  VariableName=IRB  SaveFormat=Structure With Time  SampleTime=-1
  To Workspace3 : ToWorkspace  VariableName=omega  SaveFormat=Structure With Time  SampleTime=-1
  To Workspace9 : ToWorkspace  VariableName=Mq_b  SaveFormat=Structure With Time  SampleTime=-1
  F_q : Outport
  wires:
  F/1 -> Dot Product/2, Dot Product/1, Divide/1
  Constant/1 -> Product/2
  Product/1 -> Product1/2  "n_z"
  Product1/1 -> F_q/1
  Sqrt/1 -> Product1/1, Divide/2
  Dot Product/1 -> Sqrt/1
  Atttitude Extraction/1(R_d) -> Attitude Tracker/1(R_d)
  Atttitude Extraction/2(omega_d) -> Attitude Tracker/2(omega_d)
  Atttitude Extraction/3(omega_d_dot) -> Attitude Tracker/3(omega_d_dot)
  Divide/1 -> Atttitude Extraction/1(n_d)  "n1"
  Attitude Dynamics/4(omega_b) -> To Workspace3/1, Attitude Tracker/5(omega)
  Attitude Dynamics/3(Euler) -> To Workspace1/1  "Euler"
  Attitude Dynamics/2(RBI) -> Terminator/1
  Attitude Tracker/1(Torque_in_body_frame) -> To Workspace9/1, Attitude Dynamics/1(MB)  "Mq_b"
  Attitude Dynamics/1(RIB) -> To Workspace2/1, Attitude Tracker/4(R), Product/1  "IRB"

== system TIE2019Simulation/UDE/Control_Force/h1 ==
  X : Inport
  Constant : Constant  Value=c_x
  Divide : Product  Inputs=*/
  Math Function : Math  Operator=transpose  SaturateOnIntegerOverflow=on
  Product : Product  Multiplication=Matrix(*)
  Sum : Sum  Inputs=|++
  h(X) : Outport
  wires:
  X/1 -> Divide/1, Product/2, Math Function/1
  Math Function/1 -> Product/1
  Product/1 -> Sum/1
  Constant/1 -> Sum/2
  Divide/1 -> h(X)/1
  Sum/1 -> Divide/2

== system TIE2019Simulation/UDE/Control_Force/h2 ==
  X : Inport
  Constant : Constant  Value=c_v
  Divide : Product  Inputs=*/
  Math Function : Math  Operator=transpose  SaturateOnIntegerOverflow=on
  Product : Product  Multiplication=Matrix(*)
  Sum : Sum  Inputs=|++
  h(X) : Outport
  wires:
  X/1 -> Divide/1, Product/2, Math Function/1
  Math Function/1 -> Product/1
  Product/1 -> Sum/1
  Constant/1 -> Sum/2
  Divide/1 -> h(X)/1
  Sum/1 -> Divide/2

== system TIE2019Simulation/Normal/Control_Force/Subsystem/Attitude Dynamics ==
  note: Compute payload attitude
  MB : Inport
  Constant : Constant  Value=omega_b01  VectorParams1D=off
  Constant1 : Constant  Value=invJ_B1  VectorParams1D=off
  Constant2 : Constant  Value=J  VectorParams1D=off
  Cross Matrix : Subsystem
  Integrator : Integrator  InitialConditionSource=external
  Product : Product  Multiplication=Matrix(*)
  Product1 : Product  Multiplication=Matrix(*)
  Product2 : Product  Multiplication=Matrix(*)
  Quaternion Based Attitude Calculation : Subsystem
  Sum : Sum  Inputs=|-+
  RIB : Outport
  RBI : Outport  Port=2
  Euler : Outport  Port=3
  omega_b : Outport  Port=4
  wires:
  [omega_b] -> Cross Matrix/1(A)
  Cross Matrix/1(AX) -> [omega_b_cross]
  [omega_b] -> Quaternion Based Attitude Calculation/1(OmegaBI,B)
  Quaternion Based Attitude Calculation/1(IRB) -> RIB/1
  Quaternion Based Attitude Calculation/2(BRI) -> RBI/1
  Quaternion Based Attitude Calculation/3(Euler) -> Euler/1
  Integrator/1 -> omega_b/1, [omega_b]
  Constant/1 -> Integrator/2
  Product/1 -> Integrator/1
  Constant1/1 -> Product/1
  Sum/1 -> Product/2
  MB/1 -> Sum/2
  [omega_b_cross] -> Product1/1
  Product2/1 -> Product1/2
  Constant2/1 -> Product2/1
  [omega_b] -> Product2/2
  Product1/1 -> Sum/1

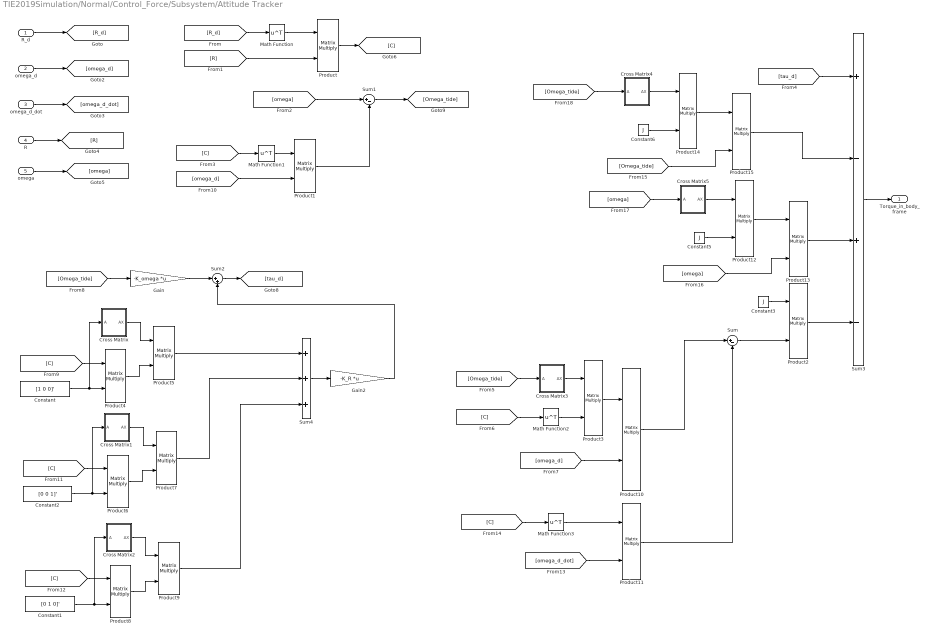
== system TIE2019Simulation/Normal/Control_Force/Subsystem/Attitude Tracker ==
  R_d : Inport
  omega_d : Inport  Port=2
  omega_d_dot : Inport  Port=3
  R : Inport  Port=4
  omega : Inport  Port=5
  Constant : Constant  Value=[1 0 0]'
  Constant1 : Constant  Value=[0 1 0]'
  Constant2 : Constant  Value=[0 0 1]'
  Constant3 : Constant  Value=J  VectorParams1D=off
  Constant5 : Constant  Value=J  VectorParams1D=off
  Constant6 : Constant  Value=J  VectorParams1D=off
  Cross Matrix : Subsystem
  Cross Matrix1 : Subsystem
  Cross Matrix2 : Subsystem
  Cross Matrix3 : Subsystem
  Cross Matrix4 : Subsystem
  Cross Matrix5 : Subsystem
  Gain : Gain  Gain=-K_omega  Multiplication=Matrix(K*u)
  Gain2 : Gain  Gain=-K_R  Multiplication=Matrix(K*u)
  Math Function{,1..3} (4 alike) : Math  Operator=transpose  SaturateOnIntegerOverflow=on
  Product{,1..15} (16 alike) : Product  Multiplication=Matrix(*)
  Sum : Sum  Inputs=|+-
  Sum1 : Sum  Inputs=|+-
  Sum2 : Sum  Inputs=|++
  Sum3 : Sum  Inputs=+-+-
  Sum4 : Sum  Inputs=+++
  Torque_in_body_frame : Outport
  wires:
  R_d/1 -> [R_d]
  omega_d/1 -> [omega_d]
  omega_d_dot/1 -> [omega_d_dot]
  [R_d] -> Math Function/1
  Math Function/1 -> Product/1
  R/1 -> [R]
  omega/1 -> [omega]
  [R] -> Product/2
  Product/1 -> [C]
  [C] -> Math Function1/1
  Math Function1/1 -> Product1/1
  [omega] -> Sum1/1
  Product1/1 -> Sum1/2
  Sum1/1 -> [Omega_tide]
  [omega_d] -> Product1/2
  Sum2/1 -> [tau_d]
  Gain/1 -> Sum2/1
  [Omega_tide] -> Gain/1
  [tau_d] -> Sum3/1
  [C] -> Product4/1
  Constant/1 -> Cross Matrix/1(A), Product4/2
  Cross Matrix/1(AX) -> Product5/1
  Product4/1 -> Product5/2
  [C] -> Product6/1
  Constant2/1 -> Cross Matrix1/1(A), Product6/2
  Cross Matrix1/1(AX) -> Product7/1
  Product6/1 -> Product7/2
  Product7/1 -> Sum4/2
  Sum4/1 -> Gain2/1
  [C] -> Product8/1
  Constant1/1 -> Cross Matrix2/1(A), Product8/2
  Cross Matrix2/1(AX) -> Product9/1
  Product8/1 -> Product9/2
  Product9/1 -> Sum4/3
  Product5/1 -> Sum4/1
  Gain2/1 -> Sum2/2
  Sum3/1 -> Torque_in_body_frame/1
  Constant3/1 -> Product2/1
  Sum/1 -> Product2/2
  [Omega_tide] -> Cross Matrix3/1(A)
  [C] -> Math Function2/1
  Cross Matrix3/1(AX) -> Product3/1
  Math Function2/1 -> Product3/2
  Product3/1 -> Product10/1
  [omega_d] -> Product10/2
  Product10/1 -> Sum/1
  [C] -> Math Function3/1
  Math Function3/1 -> Product11/1
  [omega_d_dot] -> Product11/2
  Product11/1 -> Sum/2
  Product2/1 -> Sum3/4
  Product13/1 -> Sum3/3
  Product12/1 -> Product13/1
  [omega] -> Product13/2
  [omega] -> Cross Matrix5/1(A)
  Cross Matrix5/1(AX) -> Product12/1
  Constant5/1 -> Product12/2
  Product14/1 -> Product15/1
  [Omega_tide] -> Product15/2
  [Omega_tide] -> Cross Matrix4/1(A)
  Cross Matrix4/1(AX) -> Product14/1
  Constant6/1 -> Product14/2
  Product15/1 -> Sum3/2

== system TIE2019Simulation/Normal/Control_Force/Subsystem/Atttitude Extraction ==
  n_d : Inport
  Constant1 : Constant  Value=0
  Constant2 : Constant
  Constant3 : Constant
  Derivative : Derivative
  Derivative1 : Derivative
  Display : Display
  Display1 : Display
  Math Function4 : Math  Operator=transpose  SaturateOnIntegerOverflow=on
  Product1 : Product
  Product4 : Product  Multiplication=Matrix(*)
  Saturation : Saturate  UpperLimit=10  LowerLimit=-10
  Scope{,1..3} (4 alike) : Scope
  Subsystem : Subsystem
  Switch : Switch  Criteria=u2 > Threshold  Threshold=0.99  ZeroCross=off
  Transfer Fcn1 : TransferFcn  Numerator=[5]  Denominator=[1 5]
  vee map : Subsystem
  R_d : Outport
  omega_d : Outport  Port=2
  omega_d_dot : Outport  Port=3
  wires:
  Math Function4/1 -> Product4/1
  Derivative1/1 -> Product4/2
  Product4/1 -> vee map/1(skrew symmetric matrix)
  vee map/1(phi) -> Derivative/1, Display1/1, Scope2/1, omega_d/1
  n_d/1 -> Subsystem/1(nz)  "n1"
  Constant1/1 -> Subsystem/2(psi)
  Subsystem/1(RIB_d) -> Derivative1/1, Math Function4/1, Scope3/1, R_d/1
  Constant2/1 -> Transfer Fcn1/1
  Derivative/1 -> Product1/1
  Product1/1 -> Display/1, Scope1/1, Saturation/1
  Switch/1 -> Scope/1, Product1/2
  Constant3/1 -> Switch/1
  Transfer Fcn1/1 -> Switch/2, Switch/3
  Saturation/1 -> omega_d_dot/1

== system TIE2019Simulation/UDE/Control_Force/Subsystem/Attitude Dynamics ==
  note: Compute payload attitude
  MB : Inport
  Constant : Constant  Value=omega_b01  VectorParams1D=off
  Constant1 : Constant  Value=invJ_B1  VectorParams1D=off
  Constant2 : Constant  Value=J  VectorParams1D=off
  Cross Matrix : Subsystem
  Integrator : Integrator  InitialConditionSource=external
  Product : Product  Multiplication=Matrix(*)
  Product1 : Product  Multiplication=Matrix(*)
  Product2 : Product  Multiplication=Matrix(*)
  Quaternion Based Attitude Calculation : Subsystem
  Sum : Sum  Inputs=|-+
  RIB : Outport
  RBI : Outport  Port=2
  Euler : Outport  Port=3
  omega_b : Outport  Port=4
  wires:
  [omega_b] -> Cross Matrix/1(A)
  Cross Matrix/1(AX) -> [omega_b_cross]
  [omega_b] -> Quaternion Based Attitude Calculation/1(OmegaBI,B)
  Quaternion Based Attitude Calculation/1(IRB) -> RIB/1
  Quaternion Based Attitude Calculation/2(BRI) -> RBI/1
  Quaternion Based Attitude Calculation/3(Euler) -> Euler/1
  Integrator/1 -> omega_b/1, [omega_b]
  Constant/1 -> Integrator/2
  Product/1 -> Integrator/1
  Constant1/1 -> Product/1
  Sum/1 -> Product/2
  MB/1 -> Sum/2
  [omega_b_cross] -> Product1/1
  Product2/1 -> Product1/2
  Constant2/1 -> Product2/1
  [omega_b] -> Product2/2
  Product1/1 -> Sum/1

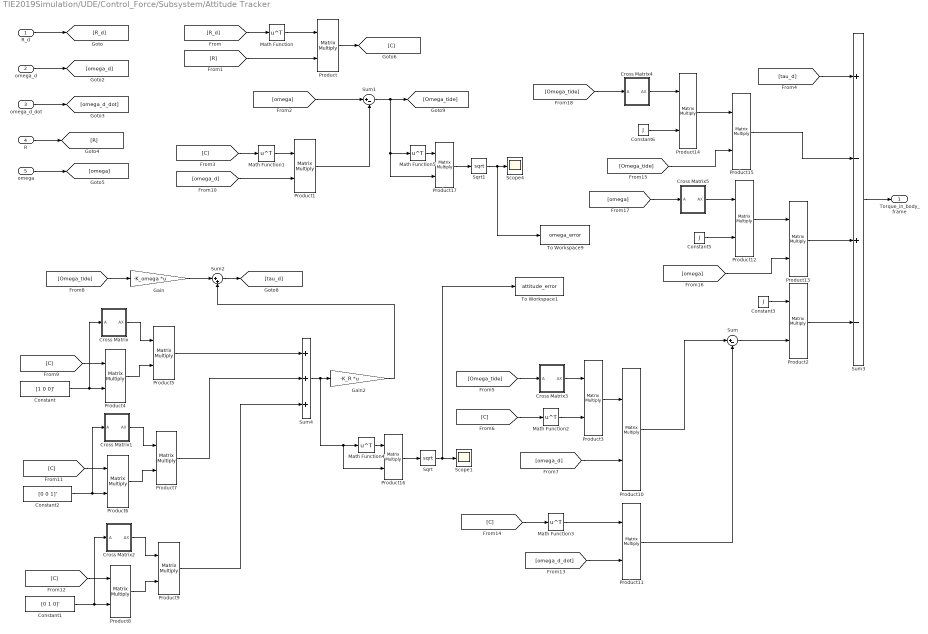
== system TIE2019Simulation/UDE/Control_Force/Subsystem/Attitude Tracker ==
  R_d : Inport
  omega_d : Inport  Port=2
  omega_d_dot : Inport  Port=3
  R : Inport  Port=4
  omega : Inport  Port=5
  Constant : Constant  Value=[1 0 0]'
  Constant1 : Constant  Value=[0 1 0]'
  Constant2 : Constant  Value=[0 0 1]'
  Constant3 : Constant  Value=J  VectorParams1D=off
  Constant5 : Constant  Value=J  VectorParams1D=off
  Constant6 : Constant  Value=J  VectorParams1D=off
  Cross Matrix : Subsystem
  Cross Matrix1 : Subsystem
  Cross Matrix2 : Subsystem
  Cross Matrix3 : Subsystem
  Cross Matrix4 : Subsystem
  Cross Matrix5 : Subsystem
  Gain : Gain  Gain=-K_omega  Multiplication=Matrix(K*u)
  Gain2 : Gain  Gain=-K_R  Multiplication=Matrix(K*u)
  Math Function{,1..5} (6 alike) : Math  Operator=transpose  SaturateOnIntegerOverflow=on
  Product{,1..17} (18 alike) : Product  Multiplication=Matrix(*)
  Scope1 : Scope
  Scope4 : Scope
  Sqrt : Sqrt  SaturateOnIntegerOverflow=on
  Sqrt1 : Sqrt  SaturateOnIntegerOverflow=on
  Sum : Sum  Inputs=|+-
  Sum1 : Sum  Inputs=|+-
  Sum2 : Sum  Inputs=|++
  Sum3 : Sum  Inputs=+-+-
  Sum4 : Sum  Inputs=+++
  To Workspace1 : ToWorkspace  VariableName=attitude_error  SampleTime=-1
  To Workspace9 : ToWorkspace  VariableName=omega_error  SampleTime=-1
  Torque_in_body_frame : Outport
  wires:
  R_d/1 -> [R_d]
  omega_d/1 -> [omega_d]
  omega_d_dot/1 -> [omega_d_dot]
  [R_d] -> Math Function/1
  Math Function/1 -> Product/1
  R/1 -> [R]
  omega/1 -> [omega]
  [R] -> Product/2
  Product/1 -> [C]
  [C] -> Math Function1/1
  Math Function1/1 -> Product1/1
  [omega] -> Sum1/1
  Product1/1 -> Sum1/2
  [omega_d] -> Product1/2
  Sum2/1 -> [tau_d]
  Gain/1 -> Sum2/1
  [Omega_tide] -> Gain/1
  [tau_d] -> Sum3/1
  [C] -> Product4/1
  Constant/1 -> Cross Matrix/1(A), Product4/2
  Cross Matrix/1(AX) -> Product5/1
  Product4/1 -> Product5/2
  [C] -> Product6/1
  Constant2/1 -> Cross Matrix1/1(A), Product6/2
  Cross Matrix1/1(AX) -> Product7/1
  Product6/1 -> Product7/2
  Product7/1 -> Sum4/2
  [C] -> Product8/1
  Constant1/1 -> Cross Matrix2/1(A), Product8/2
  Cross Matrix2/1(AX) -> Product9/1
  Product8/1 -> Product9/2
  Product9/1 -> Sum4/3
  Product5/1 -> Sum4/1
  Gain2/1 -> Sum2/2
  Sum3/1 -> Torque_in_body_frame/1
  Constant3/1 -> Product2/1
  Sum/1 -> Product2/2
  [Omega_tide] -> Cross Matrix3/1(A)
  [C] -> Math Function2/1
  Cross Matrix3/1(AX) -> Product3/1
  Math Function2/1 -> Product3/2
  Product3/1 -> Product10/1
  [omega_d] -> Product10/2
  Product10/1 -> Sum/1
  [C] -> Math Function3/1
  Math Function3/1 -> Product11/1
  [omega_d_dot] -> Product11/2
  Product11/1 -> Sum/2
  Product2/1 -> Sum3/4
  Product13/1 -> Sum3/3
  Product12/1 -> Product13/1
  [omega] -> Product13/2
  [omega] -> Cross Matrix5/1(A)
  Cross Matrix5/1(AX) -> Product12/1
  Constant5/1 -> Product12/2
  Product14/1 -> Product15/1
  [Omega_tide] -> Product15/2
  [Omega_tide] -> Cross Matrix4/1(A)
  Cross Matrix4/1(AX) -> Product14/1
  Constant6/1 -> Product14/2
  Product15/1 -> Sum3/2
  Sum4/1 -> Product16/2, Math Function4/1, Gain2/1
  Math Function4/1 -> Product16/1
  Product16/1 -> Sqrt/1
  Sqrt/1 -> To Workspace1/1, Scope1/1
  Sum1/1 -> Math Function5/1, Product17/2, [Omega_tide]
  Math Function5/1 -> Product17/1
  Product17/1 -> Sqrt1/1
  Sqrt1/1 -> To Workspace9/1, Scope4/1

== system TIE2019Simulation/UDE/Control_Force/Subsystem/Atttitude Extraction ==
  n_d : Inport
  Constant1 : Constant  Value=0
  Constant2 : Constant
  Constant3 : Constant
  Derivative : Derivative
  Derivative1 : Derivative
  Display : Display
  Display1 : Display
  Math Function4 : Math  Operator=transpose  SaturateOnIntegerOverflow=on
  Product1 : Product
  Product4 : Product  Multiplication=Matrix(*)
  Saturation : Saturate  UpperLimit=10  LowerLimit=-10
  Scope{,1..3} (4 alike) : Scope
  Subsystem : Subsystem
  Switch : Switch  Criteria=u2 > Threshold  Threshold=0.99  ZeroCross=off
  Transfer Fcn1 : TransferFcn  Numerator=[5]  Denominator=[1 5]
  vee map : Subsystem
  R_d : Outport
  omega_d : Outport  Port=2
  omega_d_dot : Outport  Port=3
  wires:
  Math Function4/1 -> Product4/1
  Derivative1/1 -> Product4/2
  Product4/1 -> vee map/1(skrew symmetric matrix)
  vee map/1(phi) -> Derivative/1, Display1/1, Scope2/1, omega_d/1
  n_d/1 -> Subsystem/1(nz)  "n1"
  Constant1/1 -> Subsystem/2(psi)
  Subsystem/1(RIB_d) -> Derivative1/1, Math Function4/1, Scope3/1, R_d/1
  Constant2/1 -> Transfer Fcn1/1
  Derivative/1 -> Product1/1
  Product1/1 -> Display/1, Scope1/1, Saturation/1
  Switch/1 -> Scope/1, Product1/2
  Constant3/1 -> Switch/1
  Transfer Fcn1/1 -> Switch/2, Switch/3
  Saturation/1 -> omega_d_dot/1
